simulink model "SimpleFOC"  (R2023a)
settings: Solver=VariableStepAuto  StartTime=0.0  StopTime=3  RelTol=1e-3
values from neighbouring files (symbols this model uses):
  Ki_id = 2*pi*BW_hz*bldc.Rs*Ts    [SystemParam.m]
  Ki_iq = 2*pi*BW_hz*bldc.Rs*Ts    [SystemParam.m]
  Kp_id = 2*pi*BW_hz*bldc.Ld    [SystemParam.m]
  Kp_iq = 2*pi*BW_hz*bldc.Lq    [SystemParam.m]
  Ts_simulink = T_pwm/20    (= 2.5e-06)    [SystemParam.m]
undefined symbols (not defined in the file or in its folder): bldc, Initial
libraries: mcbcontrolslib x9, slpidlib x2, autolibbldc x1, mcbplantlib x1
settings Model: Creator=amann  LastModifiedBy=amann
settings DebuggingCC: ParameterPrecisionLossMsg=none

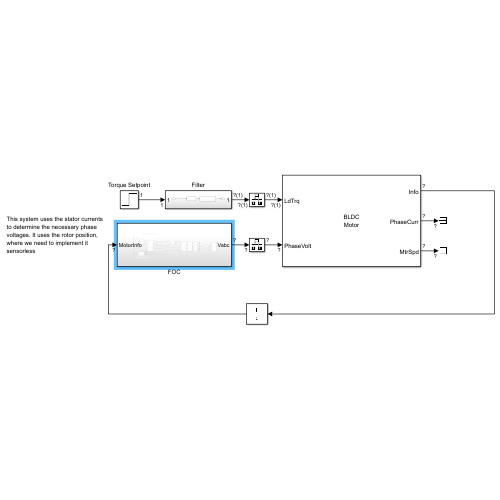
[thumbnail: Simulink's stored preview of the top-level diagram]
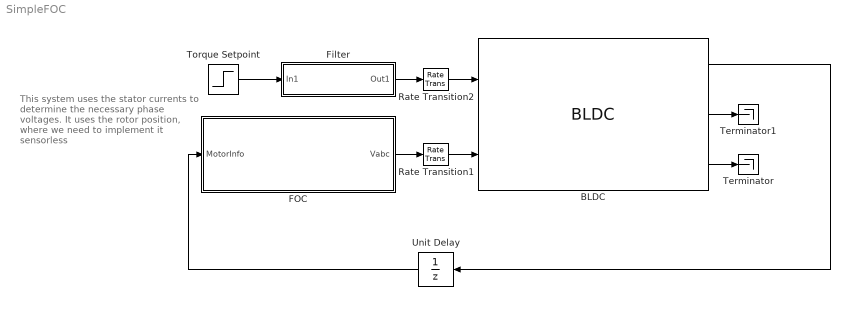
== system SimpleFOC ==
  note: This system uses the stator currents
      | to determine the necessary phase
      | voltages. It uses the rotor position,
      | where we need to implement it
      | sensorless
  BLDC : autolibbldc/BLDC  VariantControl=pmsmVariant==pmsmEnum.TorqueInput  MechInput=Torque  SimType=Discrete  BlockSampleTime=Ts_motor  p=bldc.p  Rs=bldc.Rs  Ld=bldc.Ld  Lq=bldc.Lq  Lambda=bldc.FluxPM  J=bldc.J  B=bldc.B  F=0  Id_init=Initial.bldc.ILd  Iq_init=Initial.bldc.ILq  Th_init=Initial.bldc.ITheta  Omega_init=20  RefBlkName='autolibbldc/BLDC'  aMode=5
      settings: LibrarySourceBlock=mcblib/Electrical Systems/Motors/BLDC
  FOC : Subsystem
  Filter : Subsystem
  Rate Transition1 : RateTransition  OutPortSampleTime=Ts_motor
  Rate Transition2 : RateTransition  OutPortSampleTime=Ts_motor
  Terminator : Terminator
  Terminator1 : Terminator
  Torque Setpoint : Step  Time=5  Before=Initial.Torque  After=0*bldc.T_rated  SampleTime=Ts_simulink
  Unit Delay : UnitDelay  SampleTime=-1  HasFrameUpgradeWarning=on
  wires:
  FOC/1(Vabc) -> Rate Transition1/1
  BLDC/1 -> Unit Delay/1
  Rate Transition1/1 -> BLDC/2
  BLDC/3 -> Terminator/1
  BLDC/2 -> Terminator1/1
  Rate Transition2/1 -> BLDC/1
  Unit Delay/1 -> FOC/1(MotorInfo)
  Torque Setpoint/1 -> Filter/1(In1)
  Filter/1(Out1) -> Rate Transition2/1

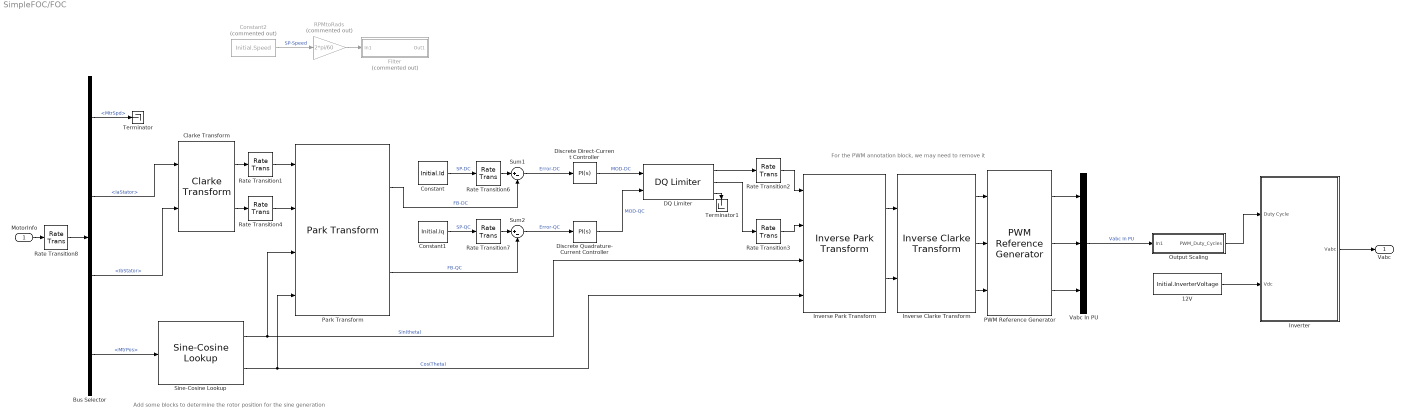
== system SimpleFOC/FOC ==
  note: Add some blocks to determine the rotor position for the sine generation
  note: For the PWM annotation block, we may need to remove it
  MotorInfo : Inport
  12V : Constant  Value=Initial.InverterVoltage
  Bus Selector : BusSelector  OutputSignals=MtrSpd,IaStator,IbStator,MtrPos
  Clarke Transform : mcbcontrolslib/Clarke Transform  VariantControl=Variant2
      settings: LibrarySourceBlock=mcblib/Controls/Math Transforms/Clarke Transform
  Constant : Constant  Value=Initial.Id  OutDataTypeStr=single
  Constant1 : Constant  Value=Initial.Iq  OutDataTypeStr=single
  Constant2 : Constant  Commented=on  Value=Initial.Speed  OutDataTypeStr=single
  DQ Limiter : mcbcontrolslib/DQ Limiter  satMethodInputType=Specify via dialog  satMethodSelected=D-Q equivalence  satLimitInputType=Specify via dialog  Vmax=1
  Discrete Direct-Current Controller : slpidlib/PID Controller  Controller=PI  Form=Parallel  TimeDomain=Continuous-time  UseExternalTs=off  SampleTime=-1  IntegratorMethod=Forward Euler  FilterMethod=Forward Euler  ControllerParametersSource=internal  P=Kp_id  I=Ki_id  UseKiTs=off  D=0  N=100  UseFilter=on  TunerSelectOption=Transfer Function Based (PID Tuner App)  InitialConditionSource=internal  InitialConditionForIntegrator=0  InitialConditionForFilter=0  DifferentiatorICPrevScaledInput=0  ExternalReset=none  TrackingMode=off  Kt=1  LimitOutput=off  SatLimitsSource=internal  UpperSaturationLimit=inf  LowerSaturationLimit=-inf  LinearizeAsGain=off  AntiWindupMode=none  Kb=1  LimitIntegrator=off  UpperIntegratorSaturationLimit=inf  LowerIntegratorSaturationLimit=-inf  POutMin=[]  POutMax=[]  IOutMin=[]  IOutMax=[]  DOutMin=[]  DOutMax=[]  NOutMin=[]  NOutMax=[]  SumOutMin=[]  SumOutMax=[]  SaturationOutMin=[]  SaturationOutMax=[]  PParamMin=[]  PParamMax=[]  IParamMin=[]  IParamMax=[]  DParamMin=[]  DParamMax=[]  NParamMin=[]  NParamMax=[]  KbParamMin=[]  KbParamMax=[]  KtParamMin=[]  KtParamMax=[]  KbOutMin=[]  KbOutMax=[]  KtOutMin=[]  KtOutMax=[]  IntegratorOutMin=[]  IntegratorOutMax=[]  FilterOutMin=[]  FilterOutMax=[]  SumI1OutMin=[]  SumI1OutMax=[]  SumI2OutMin=[]  SumI2OutMax=[]  SumI3OutMin=[]  SumI3OutMax=[]  SumI4OutMin=[]  SumI4OutMax=[]  SumDOutMin=[]  SumDOutMax=[]  DifferentiatorOutMin=[]  DifferentiatorOutMax=[]  FilterDiffOutCoefMin=[]  FilterDiffOutCoefMax=[]  ReciprocalOutMin=[]  ReciprocalOutMax=[]  SumDenOutMin=[]  SumDenOutMax=[]  SumNumOutMin=[]  SumNumOutMax=[]  DivideOutMin=[]  DivideOutMax=[]  UdiffTsProdOutMin=[]  UdiffTsProdOutMax=[]  NTsProdOutMin=[]  NTsProdOutMax=[]  UintegralTsProdOutMin=[]  UintegralTsProdOutMax=[]  UngainTsProdOutMin=[]  UngainTsProdOutMax=[]  ClampingZeroOutDataTypeStr=Inherit: Inherit via back propagation  ClampingZeroOutMin=[]  ClampingZeroOutMax=[]  FilterDenConstantOutDataTypeStr=Inherit: Inherit via back propagation  FilterDenConstantOutMin=[]  FilterDenConstantOutMax=[]  PCopyOutDataTypeStr=Inherit: Inherit via back propagation  PCopyOutMin=[]  PCopyOutMax=[]  NCopyOutDataTypeStr=Inherit: Inherit via back propagation  NCopyOutMin=[]  NCopyOutMax=[]  IntegratorContinuousStateAttributes=''  IntegratorStateMustResolveToSignalObject=off  IntegratorRTWStateStorageClass=Auto  FilterContinuousStateAttributes=''  FilterStateMustResolveToSignalObject=off  FilterRTWStateStorageClass=Auto  ParallelPVariant=InternalParameters  IdealPVariant=Disabled  IVariant=InternalParameters  DVariant=Disabled  IntegratorVariant=Continuous  SatVariant=Disabled  AWVariant=Passthrough  PCopyVariant=Disabled  TRVariant=Disabled  FdbkBlocksVariant=Forward  IdealPFdbkVariant=Disabled  SatFdbkVariant=Disabled  DerivativeFilterVariant=Disabled  NVariant=Disabled  NCopyVariant=Disabled_SignalSpec  FilterICVariant=Disabled  IntegratorICVariant=InternalICs  ExternalResetVariant=Disabled  TRSumVariant=Passthrough  SumFdbkVariant=Disabled  SumVariant=Sum_PI  TsampFilterVariant=InternalTs  TsampNgainVariant=Passthrough  TsampIntegralVariant=Disabled_SignalSpec  ExternalSaturationOutDataTypeStr=Inherit: Same as second input
      settings: LibrarySourceBlock=simulink/Discrete/Discrete PID Controller
  Discrete Quadrature-Current Controller : slpidlib/PID Controller  Controller=PI  Form=Parallel  TimeDomain=Continuous-time  UseExternalTs=off  SampleTime=-1  IntegratorMethod=Forward Euler  FilterMethod=Forward Euler  ControllerParametersSource=internal  P=Kp_iq  I=Ki_iq  UseKiTs=off  D=0  N=100  UseFilter=on  TunerSelectOption=Transfer Function Based (PID Tuner App)  InitialConditionSource=internal  InitialConditionForIntegrator=0  InitialConditionForFilter=0  DifferentiatorICPrevScaledInput=0  ExternalReset=none  TrackingMode=off  Kt=1  LimitOutput=off  SatLimitsSource=internal  UpperSaturationLimit=inf  LowerSaturationLimit=-inf  LinearizeAsGain=off  AntiWindupMode=none  Kb=1  LimitIntegrator=off  UpperIntegratorSaturationLimit=inf  LowerIntegratorSaturationLimit=-inf  POutMin=[]  POutMax=[]  IOutMin=[]  IOutMax=[]  DOutMin=[]  DOutMax=[]  NOutMin=[]  NOutMax=[]  SumOutMin=[]  SumOutMax=[]  SaturationOutMin=[]  SaturationOutMax=[]  PParamMin=[]  PParamMax=[]  IParamMin=[]  IParamMax=[]  DParamMin=[]  DParamMax=[]  NParamMin=[]  NParamMax=[]  KbParamMin=[]  KbParamMax=[]  KtParamMin=[]  KtParamMax=[]  KbOutMin=[]  KbOutMax=[]  KtOutMin=[]  KtOutMax=[]  IntegratorOutMin=[]  IntegratorOutMax=[]  FilterOutMin=[]  FilterOutMax=[]  SumI1OutMin=[]  SumI1OutMax=[]  SumI2OutMin=[]  SumI2OutMax=[]  SumI3OutMin=[]  SumI3OutMax=[]  SumI4OutMin=[]  SumI4OutMax=[]  SumDOutMin=[]  SumDOutMax=[]  DifferentiatorOutMin=[]  DifferentiatorOutMax=[]  FilterDiffOutCoefMin=[]  FilterDiffOutCoefMax=[]  ReciprocalOutMin=[]  ReciprocalOutMax=[]  SumDenOutMin=[]  SumDenOutMax=[]  SumNumOutMin=[]  SumNumOutMax=[]  DivideOutMin=[]  DivideOutMax=[]  UdiffTsProdOutMin=[]  UdiffTsProdOutMax=[]  NTsProdOutMin=[]  NTsProdOutMax=[]  UintegralTsProdOutMin=[]  UintegralTsProdOutMax=[]  UngainTsProdOutMin=[]  UngainTsProdOutMax=[]  ClampingZeroOutDataTypeStr=Inherit: Inherit via back propagation  ClampingZeroOutMin=[]  ClampingZeroOutMax=[]  FilterDenConstantOutDataTypeStr=Inherit: Inherit via back propagation  FilterDenConstantOutMin=[]  FilterDenConstantOutMax=[]  PCopyOutDataTypeStr=Inherit: Inherit via back propagation  PCopyOutMin=[]  PCopyOutMax=[]  NCopyOutDataTypeStr=Inherit: Inherit via back propagation  NCopyOutMin=[]  NCopyOutMax=[]  IntegratorContinuousStateAttributes=''  IntegratorStateMustResolveToSignalObject=off  IntegratorRTWStateStorageClass=Auto  FilterContinuousStateAttributes=''  FilterStateMustResolveToSignalObject=off  FilterRTWStateStorageClass=Auto  ParallelPVariant=InternalParameters  IdealPVariant=Disabled  IVariant=InternalParameters  DVariant=Disabled  IntegratorVariant=Continuous  SatVariant=Disabled  AWVariant=Passthrough  PCopyVariant=Disabled  TRVariant=Disabled  FdbkBlocksVariant=Forward  IdealPFdbkVariant=Disabled  SatFdbkVariant=Disabled  DerivativeFilterVariant=Disabled  NVariant=Disabled  NCopyVariant=Disabled_SignalSpec  FilterICVariant=Disabled  IntegratorICVariant=InternalICs  ExternalResetVariant=Disabled  TRSumVariant=Passthrough  SumFdbkVariant=Disabled  SumVariant=Sum_PI  TsampFilterVariant=InternalTs  TsampNgainVariant=Passthrough  TsampIntegralVariant=Disabled_SignalSpec  ExternalSaturationOutDataTypeStr=Inherit: Same as second input
      settings: LibrarySourceBlock=simulink/Discrete/Discrete PID Controller
  Filter : Subsystem  Commented=on
  Inverse Clarke Transform : mcbcontrolslib/Inverse Clarke Transform
      settings: LibrarySourceBlock=mcblib/Controls/Math Transforms/Inverse Clarke Transform
  Inverse Park Transform : mcbcontrolslib/Inverse Park Transform  AxisAlignment=D-axis
      settings: LibrarySourceBlock=mcblib/Controls/Math Transforms/Inverse Park Transform
  Inverter : Subsystem
  Output Scaling : Subsystem
  PWM Reference Generator : mcbcontrolslib/PWM Reference Generator  inSignal=Vabc  modType=SVM: space vector modulation
      settings: LibrarySourceBlock=mcblib/Controls/Math Transforms/PWM Reference Generator
  Park Transform : mcbcontrolslib/Park Transform  AxisAlignment=D-axis
      settings: LibrarySourceBlock=mcblib/Controls/Math Transforms/Park Transform
  RPMtoRads : Gain  Commented=on  Gain=2*pi/60
  Rate Transition{1..4,6..8} (7 alike) : RateTransition  InitialCondition=Ts_simulink
  Sine-Cosine Lookup : mcbcontrolslib/Sine-Cosine Lookup  AngleInput=Radians  N_points=1024
      settings: LibrarySourceBlock=mcblib/Controls/Math Transforms/Sine-Cosine Lookup
  Sum1 : Sum  Inputs=|+-
  Sum2 : Sum  Inputs=|+-
  Terminator : Terminator
  Terminator1 : Terminator
  Vabc In PU : Mux  Inputs=3
  Vabc : Outport
  wires:
  Inverse Park Transform/1 -> Inverse Clarke Transform/1
  Inverse Park Transform/2 -> Inverse Clarke Transform/2
  Inverse Clarke Transform/2 -> PWM Reference Generator/2
  Inverse Clarke Transform/1 -> PWM Reference Generator/1
  Inverse Clarke Transform/3 -> PWM Reference Generator/3
  Clarke Transform/1 -> Rate Transition1/1
  Clarke Transform/2 -> Rate Transition4/1
  Park Transform/2 -> Sum2/2  "FB-QC"
  Sine-Cosine Lookup/2 -> Park Transform/4, Inverse Park Transform/4  "Cos(Theta)"
  Sine-Cosine Lookup/1 -> Inverse Park Transform/3, Park Transform/3  "Sin(theta)"
  Rate Transition2/1 -> Inverse Park Transform/1
  Rate Transition3/1 -> Inverse Park Transform/2
  PWM Reference Generator/3 -> Vabc In PU/3
  PWM Reference Generator/2 -> Vabc In PU/2
  PWM Reference Generator/1 -> Vabc In PU/1
  MotorInfo/1 -> Rate Transition8/1
  Bus Selector/2 -> Clarke Transform/1  "<IaStator>"
  Bus Selector/3 -> Clarke Transform/2  "<IbStator>"
  Rate Transition8/1 -> Bus Selector/1
  Bus Selector/4 -> Sine-Cosine Lookup/1  "<MtrPos>"
  Constant1/1 -> Rate Transition7/1  "SP-QC"
  Constant/1 -> Rate Transition6/1  "SP-DC"
  Constant2/1 -> RPMtoRads/1  "SP-Speed"
  RPMtoRads/1 -> Filter/1(In1)
  Park Transform/1 -> Sum1/2  "FB-DC"
  Sum1/1 -> Discrete Direct-Current Controller/1  "Error-DC"
  Sum2/1 -> Discrete Quadrature-Current Controller/1  "Error-QC"
  Rate Transition7/1 -> Sum2/1
  Discrete Direct-Current Controller/1 -> DQ Limiter/1  "MOD-DC"
  Rate Transition6/1 -> Sum1/1
  Bus Selector/1 -> Terminator/1  "<MtrSpd>"
  Rate Transition1/1 -> Park Transform/1
  Rate Transition4/1 -> Park Transform/2
  DQ Limiter/3 -> Terminator1/1
  DQ Limiter/1 -> Rate Transition2/1
  Discrete Quadrature-Current Controller/1 -> DQ Limiter/2  "MOD-QC"
  DQ Limiter/2 -> Rate Transition3/1
  Vabc In PU/1 -> Output Scaling/1(In1)  "Vabc In PU"
  Output Scaling/1(PWM_Duty_Cycles) -> Inverter/1(Duty Cycle)
  12V/1 -> Inverter/2(Vdc)
  Inverter/1(Vabc) -> Vabc/1

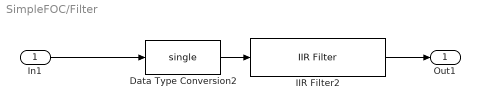
== system SimpleFOC/Filter ==
  In1 : Inport
  Data Type Conversion2 : DataTypeConversion  OutDataTypeStr=single  SaturateOnIntegerOverflow=off  RndMeth=Floor
  IIR Filter2 : mcbcontrolslib/IIR Filter  VariantControl=Low Pass Filter  VariantSelect=Low-pass  Filter_constant=0.01  advancedSettings=off  Ts=50e-6  cutOff_freq=32.1525
      settings: LibrarySourceBlock=mcblib/Signal Management/IIR Filter
  Out1 : Outport
  wires:
  Data Type Conversion2/1 -> IIR Filter2/1
  In1/1 -> Data Type Conversion2/1
  IIR Filter2/1 -> Out1/1

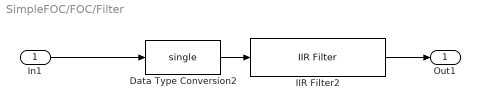
== system SimpleFOC/FOC/Filter ==
  In1 : Inport
  Data Type Conversion2 : DataTypeConversion  OutDataTypeStr=single  SaturateOnIntegerOverflow=off  RndMeth=Floor
  IIR Filter2 : mcbcontrolslib/IIR Filter  VariantControl=Low Pass Filter  VariantSelect=Low-pass  Filter_constant=0.01  advancedSettings=off  Ts=50e-6  cutOff_freq=32.1525
      settings: LibrarySourceBlock=mcblib/Signal Management/IIR Filter
  Out1 : Outport
  wires:
  Data Type Conversion2/1 -> IIR Filter2/1
  In1/1 -> Data Type Conversion2/1
  IIR Filter2/1 -> Out1/1

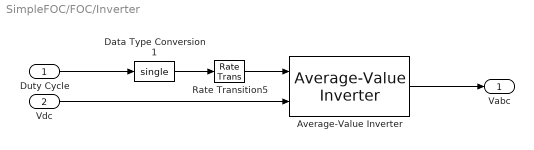
== system SimpleFOC/FOC/Inverter ==
  Duty Cycle : Inport
  Vdc : Inport  Port=2
  Average-Value Inverter : mcbplantlib/Average-Value Inverter
      settings: LibrarySourceBlock=mcblib/Electrical Systems/Inverters/Average-Value Inverter
  Data Type Conversion1 : DataTypeConversion  OutDataTypeStr=single  RndMeth=Simplest  SaturateOnIntegerOverflow=off
  Rate Transition5 : RateTransition  InitialCondition=Ts_simulink
  Vabc : Outport
  wires:
  Data Type Conversion1/1 -> Rate Transition5/1
  Duty Cycle/1 -> Data Type Conversion1/1
  Average-Value Inverter/1 -> Vabc/1
  Rate Transition5/1 -> Average-Value Inverter/1
  Vdc/1 -> Average-Value Inverter/2

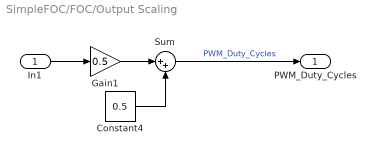
== system SimpleFOC/FOC/Output Scaling ==
  In1 : Inport
  Constant4 : Constant  Value=0.5
  Gain1 : Gain  Gain=0.5
  Sum : Sum  Inputs=|++
  PWM_Duty_Cycles : Outport
  wires:
  Gain1/1 -> Sum/1
  Constant4/1 -> Sum/2
  In1/1 -> Gain1/1
  Sum/1 -> PWM_Duty_Cycles/1  "PWM_Duty_Cycles"
